simulink model "blocks_sitl_only"  (R2017b)
settings: Solver=VariableStepAuto  StartTime=0.0  StopTime=10.0  RelTol=1e-3
settings Model: Creator=Martin  LastModifiedBy=Martin

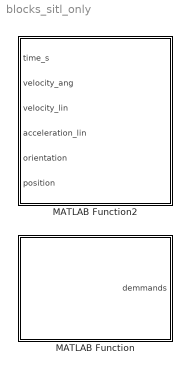
== system blocks_sitl_only ==
  MATLAB Function : MATLAB Function  TreatAsAtomicUnit=on  SystemSampleTime=0.02
  MATLAB Function2 : MATLAB Function  TreatAsAtomicUnit=on  SystemSampleTime=0.002

== matlab function blocks_sitl_only/MATLAB Function ==
  data: demmands output
function demmands = fcn()
demmands = zeros(16 ,1);
coder.extrinsic('-sync:on','simReceive');
demmands = simReceive();
end

== matlab function blocks_sitl_only/MATLAB Function2 ==
  data: time_s input; velocity_ang input; velocity_lin input; acceleration_lin input; orientation input; position input
function fcn(time_s, velocity_ang, velocity_lin, acceleration_lin, orientation, position)
coder.extrinsic('-sync:on','simSend');
simSend(time_s, velocity_ang, velocity_lin, acceleration_lin, orientation, position);
